simulink library "fordypningsprosjekt"  (Simulink 7.1)
values from neighbouring files (symbols this model uses):
  noise = variance.*randn(6,1)    [camsim3.m]
undefined symbols (not defined in the file or in its folder): bottom_signature, C_calc, ekf2, kalmanfilter, kalmanfilter2
libraries: marine_gnc x5, simulink_extras x3, vrlib x2, simulink x1
(part 2 of 2)

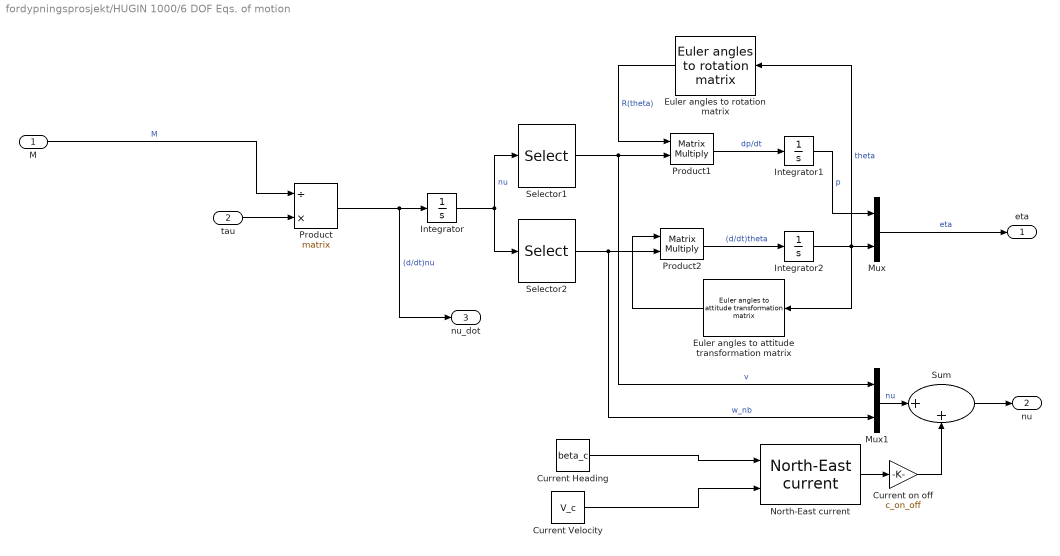
== system fordypningsprosjekt/HUGIN 1000/6 DOF Eqs. of motion ==
  M : Inport  OutDataType=sfix(16)  OutScaling=2^0
  tau : Inport  Port=2  OutDataType=sfix(16)  OutScaling=2^0
  Current Heading : Constant  Value=beta_c  OutDataType=sfix(16)  OutScaling=2^0
  Current Velocity : Constant  Value=V_c  OutDataType=sfix(16)  OutScaling=2^0
  Current on off : Gain  Gain=c_on_off  ParameterDataType=sfix(16)  ParameterScaling=2^0  OutDataType=sfix(16)  OutScaling=2^0
  Euler angles to rotation matrix : marine_gnc/Models/ Kinematics/Euler angles to rotation matrix  Orientation=left  SystemSampleTime=-1
  Euler angles to attitude transformation matrix : marine_gnc/Models/ Kinematics/Euler angles to attitude transformation matrix  Orientation=left  SystemSampleTime=-1
  Integrator : Integrator  InitialCondition=nu0
  Integrator1 : Integrator  InitialCondition=eta0(1:3)
  Integrator2 : Integrator  InitialCondition=eta0(4:6)
  Mux : Mux  Inputs=2
  Mux1 : Mux  Inputs=2
  North-East current : marine_gnc/Environment/Current/North-East current  SystemSampleTime=-1
  Product : Product  Inputs=/*  Multiplication=Matrix(*)  OutDataType=sfix(16)  OutScaling=2^0  SaturateOnIntegerOverflow=on  OutDataTypeStr=Inherit: Same as first input
  Product1 : Product  Inputs=**  Multiplication=Matrix(*)  OutDataType=sfix(16)  OutScaling=2^0  SaturateOnIntegerOverflow=on  OutDataTypeStr=Inherit: Same as first input
  Product2 : Product  Inputs=**  Multiplication=Matrix(*)  OutDataType=sfix(16)  OutScaling=2^0  SaturateOnIntegerOverflow=on  OutDataTypeStr=Inherit: Same as first input
  Selector1 : Selector  InputPortWidth=6  IndexOptions=Index vector (dialog)  Indices=[1 2 3]  OutputSizes=1
  Selector2 : Selector  InputPortWidth=6  IndexOptions=Index vector (dialog)  Indices=[4 5 6]  OutputSizes=1
  Sum : Sum  Inputs=|++  OutDataType=sfix(16)  OutScaling=2^0
  eta : Outport  OutDataType=sfix(16)  OutScaling=2^0
  nu : Outport  Port=2  OutDataType=sfix(16)  OutScaling=2^0
  nu_dot : Outport  Port=3  OutDataType=sfix(16)  OutScaling=2^0
  wires:
  Current on off/1 -> Sum/2
  Current Velocity/1 -> North-East current/2
  Current Heading/1 -> North-East current/1
  North-East current/1 -> Current on off/1
  Sum/1 -> nu/1
  Mux1/1 -> Sum/1  "nu"
  M/1 -> Product/1  "M"
  Product/1 -> nu_dot/1, Integrator/1  "(d/dt)nu"
  Integrator/1 -> Selector1/1, Selector2/1  "nu"
  Selector1/1 -> Product1/2, Mux1/1  "v"
  Selector2/1 -> Mux1/2, Product2/2  "w_nb"
  Product1/1 -> Integrator1/1  "dp/dt"
  Euler angles to rotation matrix/1 -> Product1/1  "R(theta)"
  Product2/1 -> Integrator2/1  "(d/dt)theta"
  Integrator2/1 -> Mux/2, Euler angles to rotation matrix/1, Euler angles to attitude transformation matrix/1  "theta"
  Integrator1/1 -> Mux/1  "p"
  Mux/1 -> eta/1  "eta"
  Euler angles to attitude transformation matrix/1 -> Product2/1
  tau/1 -> Product/2

== system fordypningsprosjekt/HUGIN 1000/coriolis  forces ==
  nu : Inport  OutDataType=sfix(16)  OutScaling=2^0
  Coriolis : MATLABFcn  MATLABFcn=C_calc(u)  OutputDimensions=[6,6]  Output1D=off
  Product : Product  Multiplication=Matrix(*)  OutDataType=sfix(16)  OutScaling=2^0  RndMeth=Zero
  C(nu)*nu : Outport  OutDataType=sfix(16)  OutScaling=2^0
  wires:
  Product/1 -> C(nu)*nu/1
  Coriolis/1 -> Product/1
  nu/1 -> Coriolis/1, Product/2

== system fordypningsprosjekt/HUGIN 1000/damping ==
  nu : Inport  OutDataType=sfix(16)  OutScaling=2^0
  Abs : Abs  OutDataType=sfix(16)  OutScaling=2^0
  D_nl : Constant  Value=[Xuu 0 0 0 0 0; 0 0 0 0 0 0; 0 0 0 0 0 0; 0 0 0 0 0 0; 0 0 0 0 0 0; 0 0 0 0 0 0]  OutDataType=sfix(16)  OutScaling=2^0
  Damping : Constant  Value=D  OutDataType=sfix(16)  OutScaling=2^0
  Product : Product  OutDataType=sfix(16)  OutScaling=2^0  RndMeth=Zero
  Product1 : Product  Multiplication=Matrix(*)  OutDataType=sfix(16)  OutScaling=2^0  RndMeth=Zero
  Selector : Selector  Orientation=up  InputPortWidth=6  IndexOptions=Index vector (dialog)  Indices=[1]  OutputSizes=1
  Sum : Sum  Inputs=|--  OutDataType=sfix(16)  OutScaling=2^0
  D(nu)*nu : Outport  OutDataType=sfix(16)  OutScaling=2^0
  wires:
  Selector/1 -> Abs/1
  Product1/1 -> D(nu)*nu/1
  Sum/1 -> Product1/1
  Abs/1 -> Product/2
  D_nl/1 -> Product/1
  nu/1 -> Selector/1, Product1/2
  Product/1 -> Sum/1
  Damping/1 -> Sum/2

== system fordypningsprosjekt/HUGIN 1000/restoring forces ==
  eta : Inport  OutDataType=sfix(16)  OutScaling=2^0
  Constant : Constant  Value=0  OutDataType=sfix(16)  OutScaling=2^0
  Demux : Demux  Outputs=6
  Mux : Mux  Inputs=6
  Product : Product  OutDataType=sfix(16)  OutScaling=2^0  RndMeth=Zero
  Terminator{,1..3} (4 alike) : Terminator
  cos theta : Trigonometry  Operator=cos
  sin fi : Trigonometry
  sin theta : Trigonometry
  zg*W : Gain  Gain=W*zg  ParameterDataType=sfix(16)  ParameterScaling=2^0  OutDataType=sfix(16)  OutScaling=2^0
  zg*W1 : Gain  Gain=W*zg  ParameterDataType=sfix(16)  ParameterScaling=2^0  OutDataType=sfix(16)  OutScaling=2^0
  g(eta) : Outport  OutDataType=sfix(16)  OutScaling=2^0
  wires:
  Demux/3 -> Terminator3/1
  Demux/2 -> Terminator2/1
  Demux/1 -> Terminator1/1
  Demux/6 -> Terminator/1
  Constant/1 -> Mux/6, Mux/3, Mux/2, Mux/1
  zg*W/1 -> Mux/4
  zg*W1/1 -> Mux/5
  Mux/1 -> g(eta)/1
  sin theta/1 -> zg*W1/1
  Product/1 -> zg*W/1
  sin fi/1 -> Product/1
  cos theta/1 -> Product/2
  Demux/5 -> sin theta/1, cos theta/1
  Demux/4 -> sin fi/1
  eta/1 -> Demux/1

== matlab function Switching logic ==
  data: u input double; y output double; psi_d input double; eta input double; nu input double; t input double; output input double
function y = fcn(u, psi_d, eta , nu ,t, output)
% This block supports the Embedded MATLAB subset.
% See the help menu for details. 

persistent temp

if isempty(temp)
    temp = 0;
end

xi1 = u(1);
yi1 = u(2);
xi2 = u(3);
yi2 = u(4);
xi3 = u(5);
yi3 = u(6);

beta = atan2(nu(2), sqrt(nu(1)^2 + nu(2)^2));

    if output == 1    
        if xi1 >= eta(1)
            temp = atan2((yi1),(xi1)) + beta;
        else
            temp = atan2((yi3), (xi3)) + beta;
        end
     else
         temp = psi_d;  
    end   
    
y = temp;
